simulink model "Filter"  (R2020b)
settings: Solver=FixedStepDiscrete  StartTime=0.0  StopTime=1  RelTol=1e-3
settings Model: Creator=abhin  LastModifiedBy=abhin
settings DataIOCC: ExternalInput=[t,u]  SaveFormat=Array

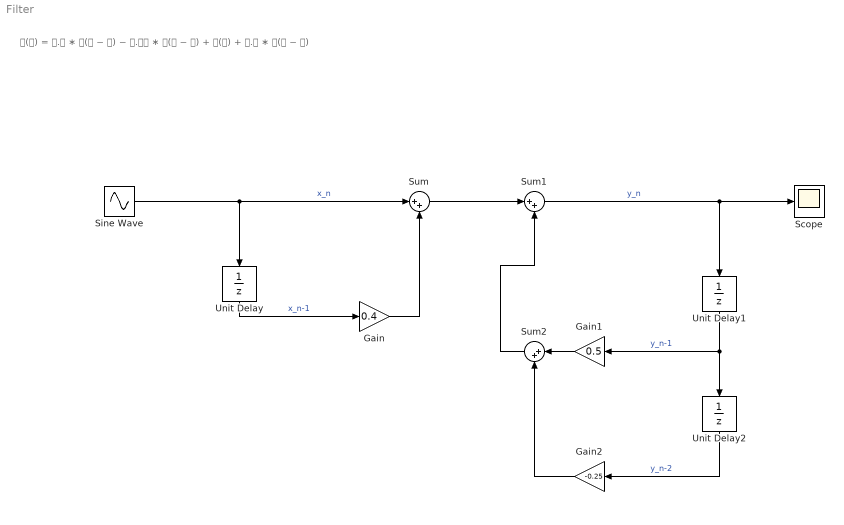
== system Filter ==
  note: 𝐲(𝐧) = 𝟎.𝟓 ∗ 𝐲(𝐧 − 𝟏) − 𝟎.𝟐𝟓 ∗ 𝐲(𝐧 − 𝟐) + 𝐱(𝐧) + 𝟎.𝟒 ∗ 𝐱(𝐧 − 𝟏)
  Gain : Gain  Gain=0.4
  Gain1 : Gain  Gain=0.5
  Gain2 : Gain  Gain=-0.25
  Scope : Scope
  Sine Wave : Sin  Amplitude=5  Frequency=2*pi*50  SampleTime=0.001
  Sum : Sum  Inputs=|++
  Sum1 : Sum  Inputs=|++
  Sum2 : Sum  Inputs=|++
  Unit Delay : UnitDelay  SampleTime=-1  HasFrameUpgradeWarning=on
  Unit Delay1 : UnitDelay  SampleTime=-1  HasFrameUpgradeWarning=on
  Unit Delay2 : UnitDelay  SampleTime=-1  HasFrameUpgradeWarning=on
  wires:
  Sine Wave/1 -> Unit Delay/1, Sum/1  "x_n"
  Unit Delay/1 -> Gain/1  "x_n-1"
  Gain/1 -> Sum/2
  Unit Delay1/1 -> Gain1/1, Unit Delay2/1  "y_n-1"
  Unit Delay2/1 -> Gain2/1  "y_n-2"
  Sum/1 -> Sum1/1
  Gain1/1 -> Sum2/1
  Gain2/1 -> Sum2/2
  Sum2/1 -> Sum1/2
  Sum1/1 -> Scope/1, Unit Delay1/1  "y_n"
